simulink model "simulink model"  (R2018b)
settings: Solver=VariableStepAuto  StartTime=0.0  StopTime=2.0  RelTol=1e-3
undefined symbols (not defined in the file): sigbuilder_block
settings Model: Creator=Aditya's HP Omen 15  LastModifiedBy=Aditya's HP Omen 15

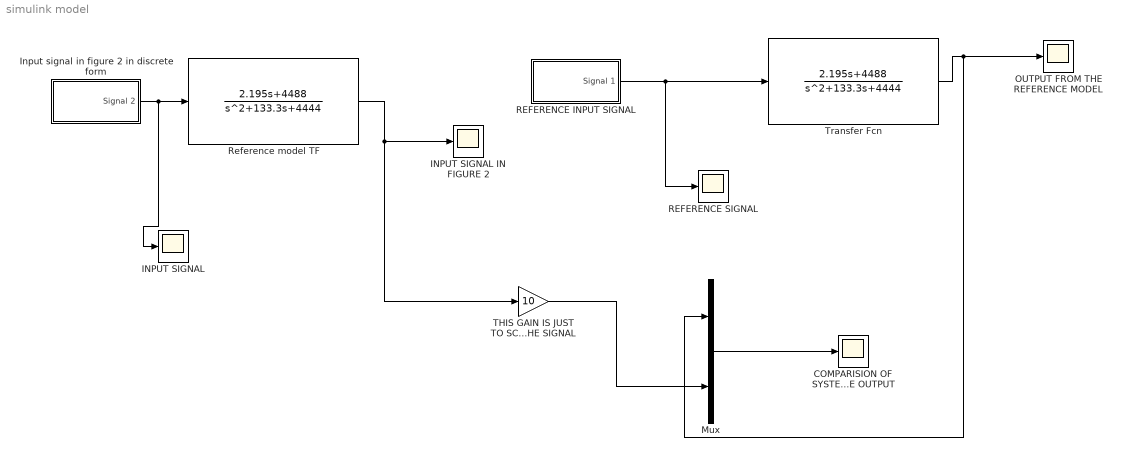
== system simulink model ==
  " OUTPUT FROM THE REFERENCE MODEL" : Scope
  COMPARISION OF SYSTEM OUTPUT AND MODEL REFERENCE OUTPUT : Scope
  INPUT SIGNAL : Scope
  INPUT SIGNAL IN FIGURE 2 : Scope
  Input signal in figure 2 in discrete form : Subsystem  Tag=STV Subsys  LoadFcn=sigbuilder_block('load');  StartFcn=sigbuilder_block('start');  StopFcn=sigbuilder_block('stop');  ClipboardFcn=sigbuilder_block('clipboard');  mask(Sigbuilder block){tuvar=[0:10]}
      mask help: Simulink:masks:SigbuilderBlock_MD
      mask init:
      | if ~strcmp(get_param(bdroot(gcbh),'SimulationStatus'),'stopped') tuvar = sigbuilder_block('maskInit'); end
      settings: CopyFcn=sigbuilder_block('copy');  DeleteFcn=sigbuilder_block('delete');  ModelCloseFcn=sigbuilder_block('modelClose');  PreSaveFcn=sigbuilder_block('preSave');  PauseFcn=sigbuilder_block('pause');  ContinueFcn=sigbuilder_block('continue');  NameChangeFcn=sigbuilder_block('namechange');  OpenFcn=sigbuilder_block('open',[368.4 108.6 550.8 361.2 ]);  CloseFcn=sigbuilder_block('close');
      mask Display: plot(0, 0, 100, 100,[2, 2, 32, 32, 2], [68, 8, 8, 68, 68],[32, 2], [38, 38], [32, 19, 2],[53, 60, 44], [32, 17, 17, 2],[16, 16, 31, 31]);txt = getActiveGroup(gcbh);text(2, 100, txt,'verticalAlignment', 'top');
  Mux : Mux  Inputs=2
  REFERENCE INPUT SIGNAL : Subsystem  Tag=STV Subsys  LoadFcn=sigbuilder_block('load');  StartFcn=sigbuilder_block('start');  StopFcn=sigbuilder_block('stop');  ClipboardFcn=sigbuilder_block('clipboard');  mask(Sigbuilder block){tuvar=[0:10]}
      mask help: Simulink:masks:SigbuilderBlock_MD
      mask init:
      | if ~strcmp(get_param(bdroot(gcbh),'SimulationStatus'),'stopped') tuvar = sigbuilder_block('maskInit'); end
      settings: CopyFcn=sigbuilder_block('copy');  DeleteFcn=sigbuilder_block('delete');  ModelCloseFcn=sigbuilder_block('modelClose');  PreSaveFcn=sigbuilder_block('preSave');  PauseFcn=sigbuilder_block('pause');  ContinueFcn=sigbuilder_block('continue');  NameChangeFcn=sigbuilder_block('namechange');  OpenFcn=sigbuilder_block('open',[-10.2 95.4 550.8 361.2 ]);  CloseFcn=sigbuilder_block('close');
      mask Display: plot(0, 0, 100, 100,[2, 2, 32, 32, 2], [68, 8, 8, 68, 68],[32, 2], [38, 38], [32, 19, 2],[53, 60, 44], [32, 17, 17, 2],[16, 16, 31, 31]);txt = getActiveGroup(gcbh);text(2, 100, txt,'verticalAlignment', 'top');
  "REFERENCE SIGNAL " : Scope
  Reference model TF : TransferFcn  Numerator=[2.195 4488]  Denominator=[1 133.3 4444]
  THIS GAIN IS JUST TO SCALE UP THE SIGNAL : Gain  Gain=10
  Transfer Fcn : TransferFcn  Numerator=[2.195 4488]  Denominator=[1 133.3 4444]
  wires:
  Transfer Fcn/1 -> Mux/1, " OUTPUT FROM THE REFERENCE MODEL"/1
  REFERENCE INPUT SIGNAL/1(Signal 1) -> "REFERENCE SIGNAL "/1, Transfer Fcn/1
  Input signal in figure 2 in discrete form/1(Signal 2) -> INPUT SIGNAL/1, Reference model TF/1
  Reference model TF/1 -> THIS GAIN IS JUST TO SCALE UP THE SIGNAL/1, INPUT SIGNAL IN FIGURE 2/1
  Mux/1 -> COMPARISION OF SYSTEM OUTPUT AND MODEL REFERENCE OUTPUT/1
  THIS GAIN IS JUST TO SCALE UP THE SIGNAL/1 -> Mux/2

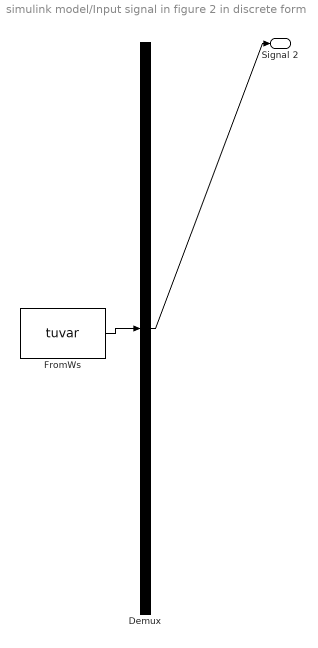
== system simulink model/Input signal in figure 2 in discrete form ==
  Demux : Demux  Tag=STV Demux  Outputs=1
  FromWs : FromWorkspace  Tag=STV FromWs  VariableName=tuvar  SampleTime=0
      SigBuilderData=|
      | common.afterFinalStr = 'Extrapolate'
      | common.sampleTime = 0
      | dataSet.timeRange = [0 10]
      | dataSet.name = 'Group 1'
      | sbobj.Groups.Name = 'Group 1'
      | sbobj.Groups.Signals.Name = 'Signal 2'
      | sbobj.Groups.Signals.XData = [0 0.05 0.15 0.23 0.4 0.5 0.6 0.7 0.8 0.9 1 1.04 1.11 1.21 1.28 1.5 1.55 1.63 1.7 1.9 10]
      | sbobj.Groups.Signals.YData = [0 20 8 10.8 10 10 20 13 15 15 15 6.2 11 9.2 10 10 20 13 15 15 15]
  Signal 2 : Outport  Tag=STV Outport
  wires:
  FromWs/1 -> Demux/1
  Demux/1 -> Signal 2/1

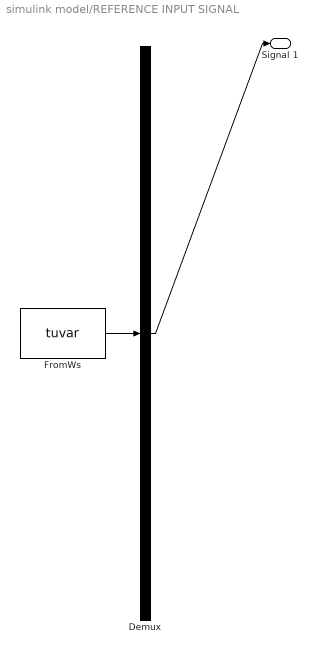
== system simulink model/REFERENCE INPUT SIGNAL ==
  Demux : Demux  Tag=STV Demux  Outputs=1
  FromWs : FromWorkspace  Tag=STV FromWs  VariableName=tuvar  SampleTime=0
      SigBuilderData=|
      | common.afterFinalStr = 'Extrapolate'
      | common.sampleTime = 0
      | dataSet.timeRange = [0 10]
      | dataSet.name = 'r(k)'
      | sbobj.Groups.Name = 'r(k)'
      | sbobj.Groups.Signals.Name = 'Signal 1'
      | sbobj.Groups.Signals.XData = [0 0.1 0.2 0.3 0.4 0.5 0.6 0.7 0.8 0.9 1 1.1 1.2 1.3 1.4 1.5 1.6 1.7 1.8 1.9 10]
      | sbobj.Groups.Signals.YData = [0 100 100 100 100 100 150 150 150 150 150 100 100 100 100 100 150 150 150 150 150]
  Signal 1 : Outport  Tag=STV Outport
  wires:
  FromWs/1 -> Demux/1
  Demux/1 -> Signal 1/1
